simulink model "EDE"  (R2024a)
settings: Solver=VariableStepAuto  StartTime=0.0  StopTime=10  RelTol=1e-3
settings Model: Creator=ansm3  LastModifiedBy=ansm3

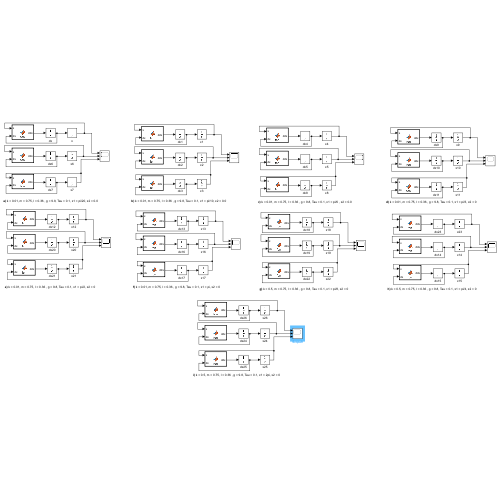
[thumbnail: Simulink's stored preview of the top-level diagram]
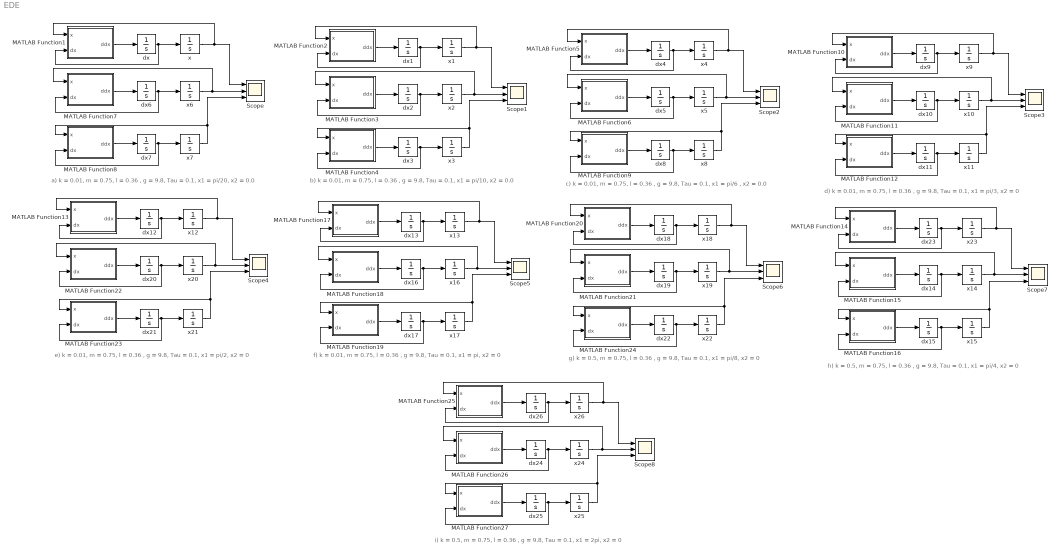
== system EDE ==
  note: a) k = 0.01, m = 0.75, l = 0.36 , g = 9.8, Tau = 0.1, x1 = pi/20, x2 = 0.0
  note: b) k = 0.01, m = 0.75, l = 0.36 , g = 9.8, Tau = 0.1, x1 = pi/10, x2 = 0.0
  note: c) k = 0.01, m = 0.75, l = 0.36 , g = 9.8, Tau = 0.1, x1 = pi/6 , x2 = 0.0
  note: d) k = 0.01, m = 0.75, l = 0.36 , g = 9.8, Tau = 0.1, x1 = pi/3, x2 = 0
  note: e) k = 0.01, m = 0.75, l = 0.36 , g = 9.8, Tau = 0.1, x1 = pi/2, x2 = 0
  note: g) k = 0.5, m = 0.75, l = 0.36 , g = 9.8, Tau = 0.1, x1 = pi/8, x2 = 0
  note: h) k = 0.5, m = 0.75, l = 0.36 , g = 9.8, Tau = 0.1, x1 = pi/4, x2 = 0
  note: f) k = 0.01, m = 0.75, l = 0.36 , g = 9.8, Tau = 0.1, x1 = pi, x2 = 0
  note: i) k = 0.5, m = 0.75, l = 0.36 , g = 9.8, Tau = 0.1, x1 = 2pi, x2 = 0
  MATLAB Function1 : MATLAB Function  TreatAsAtomicUnit=on
  MATLAB Function10 : MATLAB Function  TreatAsAtomicUnit=on
  MATLAB Function11 : MATLAB Function  TreatAsAtomicUnit=on
  MATLAB Function12 : MATLAB Function  TreatAsAtomicUnit=on
  MATLAB Function13 : MATLAB Function  TreatAsAtomicUnit=on
  MATLAB Function14 : MATLAB Function  TreatAsAtomicUnit=on
  MATLAB Function15 : MATLAB Function  TreatAsAtomicUnit=on
  MATLAB Function16 : MATLAB Function  TreatAsAtomicUnit=on
  MATLAB Function17 : MATLAB Function  TreatAsAtomicUnit=on
  MATLAB Function18 : MATLAB Function  TreatAsAtomicUnit=on
  MATLAB Function19 : MATLAB Function  TreatAsAtomicUnit=on
  MATLAB Function2 : MATLAB Function  TreatAsAtomicUnit=on
  MATLAB Function20 : MATLAB Function  TreatAsAtomicUnit=on
  MATLAB Function21 : MATLAB Function  TreatAsAtomicUnit=on
  MATLAB Function22 : MATLAB Function  TreatAsAtomicUnit=on
  MATLAB Function23 : MATLAB Function  TreatAsAtomicUnit=on
  MATLAB Function24 : MATLAB Function  TreatAsAtomicUnit=on
  MATLAB Function25 : MATLAB Function  TreatAsAtomicUnit=on
  MATLAB Function26 : MATLAB Function  TreatAsAtomicUnit=on
  MATLAB Function27 : MATLAB Function  TreatAsAtomicUnit=on
  MATLAB Function3 : MATLAB Function  TreatAsAtomicUnit=on
  MATLAB Function4 : MATLAB Function  TreatAsAtomicUnit=on
  MATLAB Function5 : MATLAB Function  TreatAsAtomicUnit=on
  MATLAB Function6 : MATLAB Function  TreatAsAtomicUnit=on
  MATLAB Function7 : MATLAB Function  TreatAsAtomicUnit=on
  MATLAB Function8 : MATLAB Function  TreatAsAtomicUnit=on
  MATLAB Function9 : MATLAB Function  TreatAsAtomicUnit=on
  Scope{,1..8} (9 alike) : Scope  NumInputPorts=3
  dx{,1..26} (27 alike) : Integrator  ContinuousStateAttributes="\"dx\""
  x : Integrator  InitialCondition=pi/20
  x1 : Integrator  InitialCondition=pi/10
  x10 : Integrator  InitialCondition=pi/3
  x11 : Integrator  InitialCondition=pi/3
  x12 : Integrator  InitialCondition=pi/2
  x13 : Integrator  InitialCondition=pi
  x14 : Integrator  InitialCondition=pi/4
  x15 : Integrator  InitialCondition=pi/4
  x16 : Integrator  InitialCondition=pi
  x17 : Integrator  InitialCondition=pi
  x18 : Integrator  InitialCondition=pi/8
  x19 : Integrator  InitialCondition=pi/8
  x2 : Integrator  InitialCondition=pi/10
  x20 : Integrator  InitialCondition=pi/2
  x21 : Integrator  InitialCondition=pi/2
  x22 : Integrator  InitialCondition=pi/8
  x23 : Integrator  InitialCondition=pi/4
  x24 : Integrator  InitialCondition=2*pi
  x25 : Integrator  InitialCondition=2*pi
  x26 : Integrator  InitialCondition=2*pi
  x3 : Integrator  InitialCondition=pi/10
  x4 : Integrator  InitialCondition=pi/6
  x5 : Integrator  InitialCondition=pi/6
  x6 : Integrator  InitialCondition=pi/20
  x7 : Integrator  InitialCondition=pi/20
  x8 : Integrator  InitialCondition=pi/6
  x9 : Integrator  InitialCondition=pi/3
  wires:
  dx/1 -> x/1, MATLAB Function1/2(dx)
  MATLAB Function1/1(ddx) -> dx/1
  x/1 -> Scope/1, MATLAB Function1/1(x)
  dx6/1 -> x6/1, MATLAB Function7/2(dx)
  MATLAB Function7/1(ddx) -> dx6/1
  x6/1 -> Scope/2, MATLAB Function7/1(x)
  MATLAB Function8/1(ddx) -> dx7/1
  dx7/1 -> x7/1, MATLAB Function8/2(dx)
  x7/1 -> Scope/3, MATLAB Function8/1(x)
  x2/1 -> Scope1/2, MATLAB Function3/1(x)
  MATLAB Function3/1(ddx) -> dx2/1
  dx2/1 -> x2/1, MATLAB Function3/2(dx)
  MATLAB Function4/1(ddx) -> dx3/1
  dx3/1 -> x3/1, MATLAB Function4/2(dx)
  dx1/1 -> x1/1, MATLAB Function2/2(dx)
  x3/1 -> Scope1/3, MATLAB Function4/1(x)
  x1/1 -> Scope1/1, MATLAB Function2/1(x)
  MATLAB Function2/1(ddx) -> dx1/1
  dx8/1 -> x8/1, MATLAB Function9/2(dx)
  dx5/1 -> x5/1, MATLAB Function6/2(dx)
  MATLAB Function9/1(ddx) -> dx8/1
  MATLAB Function6/1(ddx) -> dx5/1
  dx4/1 -> x4/1, MATLAB Function5/2(dx)
  x8/1 -> Scope2/3, MATLAB Function9/1(x)
  MATLAB Function5/1(ddx) -> dx4/1
  x4/1 -> Scope2/1, MATLAB Function5/1(x)
  x5/1 -> Scope2/2, MATLAB Function6/1(x)
  x11/1 -> Scope3/3, MATLAB Function12/1(x)
  x9/1 -> Scope3/1, MATLAB Function10/1(x)
  MATLAB Function10/1(ddx) -> dx9/1
  x10/1 -> Scope3/2, MATLAB Function11/1(x)
  dx9/1 -> x9/1, MATLAB Function10/2(dx)
  dx11/1 -> x11/1, MATLAB Function12/2(dx)
  MATLAB Function11/1(ddx) -> dx10/1
  MATLAB Function12/1(ddx) -> dx11/1
  dx10/1 -> x10/1, MATLAB Function11/2(dx)
  x20/1 -> Scope4/2, MATLAB Function22/1(x)
  dx14/1 -> x14/1, MATLAB Function15/2(dx)
  MATLAB Function15/1(ddx) -> dx14/1
  dx15/1 -> x15/1, MATLAB Function16/2(dx)
  MATLAB Function16/1(ddx) -> dx15/1
  x15/1 -> Scope7/3, MATLAB Function16/1(x)
  x14/1 -> Scope7/2, MATLAB Function15/1(x)
  MATLAB Function14/1(ddx) -> dx23/1
  MATLAB Function20/1(ddx) -> dx18/1
  dx16/1 -> x16/1, MATLAB Function18/2(dx)
  MATLAB Function19/1(ddx) -> dx17/1
  x23/1 -> Scope7/1, MATLAB Function14/1(x)
  dx23/1 -> x23/1, MATLAB Function14/2(dx)
  MATLAB Function18/1(ddx) -> dx16/1
  dx13/1 -> x13/1, MATLAB Function17/2(dx)
  x17/1 -> Scope5/3, MATLAB Function19/1(x)
  x19/1 -> Scope6/2, MATLAB Function21/1(x)
  MATLAB Function17/1(ddx) -> dx13/1
  x13/1 -> Scope5/1, MATLAB Function17/1(x)
  x22/1 -> Scope6/3, MATLAB Function24/1(x)
  MATLAB Function21/1(ddx) -> dx19/1
  MATLAB Function24/1(ddx) -> dx22/1
  MATLAB Function22/1(ddx) -> dx20/1
  dx20/1 -> x20/1, MATLAB Function22/2(dx)
  dx17/1 -> x17/1, MATLAB Function19/2(dx)
  dx21/1 -> x21/1, MATLAB Function23/2(dx)
  MATLAB Function23/1(ddx) -> dx21/1
  x16/1 -> Scope5/2, MATLAB Function18/1(x)
  dx12/1 -> x12/1, MATLAB Function13/2(dx)
  dx22/1 -> x22/1, MATLAB Function24/2(dx)
  x21/1 -> Scope4/3, MATLAB Function23/1(x)
  x18/1 -> Scope6/1, MATLAB Function20/1(x)
  MATLAB Function13/1(ddx) -> dx12/1
  dx19/1 -> x19/1, MATLAB Function21/2(dx)
  x12/1 -> Scope4/1, MATLAB Function13/1(x)
  dx18/1 -> x18/1, MATLAB Function20/2(dx)
  MATLAB Function27/1(ddx) -> dx25/1
  MATLAB Function26/1(ddx) -> dx24/1
  dx24/1 -> x24/1, MATLAB Function26/2(dx)
  dx25/1 -> x25/1, MATLAB Function27/2(dx)
  x25/1 -> Scope8/3, MATLAB Function27/1(x)
  dx26/1 -> x26/1, MATLAB Function25/2(dx)
  x26/1 -> Scope8/1, MATLAB Function25/1(x)
  x24/1 -> Scope8/2, MATLAB Function26/1(x)
  MATLAB Function25/1(ddx) -> dx26/1

== matlab function EDE/MATLAB Function13 ==
  data: x input; ddx output; dx input
function ddx = fcn(x, dx)

k=0.01;
l=0.36;
g=9.8;
a=l/2;

m=0.75;
J=(4/3)*(m*a^2);
tao=0.1;

ddx=(tao/J) - ((k*dx)/J) - ((m*g*a*x)/J);

== matlab function EDE/MATLAB Function14 ==
  data: x input; ddx output; dx input
function ddx = fcn(x, dx)

k=0.5;
l=0.36;
g=9.8;
a=l/2;

m=0.75;
J=(4/3)*(m*a^2);
tao=0.1;

ddx=(tao/J) - ((k*dx)/J) - ((m*g*a*x)/J);

== matlab function EDE/MATLAB Function15 ==
  data: x input; ddx output; dx input
function ddx = fcn(x, dx)

k=0.5;
l=0.36;
g=9.8;
a=l/2;

m=0.75;
J=(4/3)*(m*a^2);
tao=0.1;

ddx=(tao/J) - ((k*dx)/J) - ((m*g*a*sin(x))/J);

== matlab function EDE/MATLAB Function16 ==
  data: x input; ddx output; dx input
function ddx = fcn(x, dx)

k=0.5;
l=0.36;
g=9.8;
a=l/2;

m=0.75;
J=(4/3)*(m*a^2);
tao=0.1;

ddx=(tao/J) - ((k*dx)/J) - ((m*g*a*cos(x))/J);

== matlab function EDE/MATLAB Function17 ==
  data: x input; ddx output; dx input
function ddx = fcn(x, dx)

k=0.01;
l=0.36;
g=9.8;
a=l/2;

m=0.75;
J=(4/3)*(m*a^2);
tao=0.1;

ddx=(tao/J) - ((k*dx)/J) - ((m*g*a*x)/J);

== matlab function EDE/MATLAB Function18 ==
  data: x input; ddx output; dx input
function ddx = fcn(x, dx)

k=0.01;
l=0.36;
g=9.8;
a=l/2;

m=0.75;
J=(4/3)*(m*a^2);
tao=0.1;

ddx=(tao/J) - ((k*dx)/J) - ((m*g*a*sin(x))/J);

== matlab function EDE/MATLAB Function19 ==
  data: x input; ddx output; dx input
function ddx = fcn(x, dx)

k=0.01;
l=0.36;
g=9.8;
a=l/2;

m=0.75;
J=(4/3)*(m*a^2);
tao=0.1;

ddx=(tao/J) - ((k*dx)/J) - ((m*g*a*cos(x))/J);

== matlab function EDE/MATLAB Function2 ==
  data: x input; ddx output; dx input
function ddx = fcn(x, dx)

k=0.01;
l=0.36;
g=9.8;
a=l/2;

m=0.75;
J=(4/3)*(m*a^2);
tao=0.1;

ddx=(tao/J) - ((k*dx)/J) - ((m*g*a*x)/J);

== matlab function EDE/MATLAB Function20 ==
  data: x input; ddx output; dx input
function ddx = fcn(x, dx)

k=0.5;
l=0.36;
g=9.8;
a=l/2;

m=0.75;
J=(4/3)*(m*a^2);
tao=0.1;

ddx=(tao/J) - ((k*dx)/J) - ((m*g*a*x)/J);

== matlab function EDE/MATLAB Function21 ==
  data: x input; ddx output; dx input
function ddx = fcn(x, dx)

k=0.5;
l=0.36;
g=9.8;
a=l/2;

m=0.75;
J=(4/3)*(m*a^2);
tao=0.1;

ddx=(tao/J) - ((k*dx)/J) - ((m*g*a*sin(x))/J);

== matlab function EDE/MATLAB Function22 ==
  data: x input; ddx output; dx input
function ddx = fcn(x, dx)

k=0.01;
l=0.36;
g=9.8;
a=l/2;

m=0.75;
J=(4/3)*(m*a^2);
tao=0.1;

ddx=(tao/J) - ((k*dx)/J) - ((m*g*a*sin(x))/J);

== matlab function EDE/MATLAB Function23 ==
  data: x input; ddx output; dx input
function ddx = fcn(x, dx)

k=0.01;
l=0.36;
g=9.8;
a=l/2;

m=0.75;
J=(4/3)*(m*a^2);
tao=0.1;

ddx=(tao/J) - ((k*dx)/J) - ((m*g*a*cos(x))/J);

== matlab function EDE/MATLAB Function24 ==
  data: x input; ddx output; dx input
function ddx = fcn(x, dx)

k=0.5;
l=0.36;
g=9.8;
a=l/2;

m=0.75;
J=(4/3)*(m*a^2);
tao=0.1;

ddx=(tao/J) - ((k*dx)/J) - ((m*g*a*cos(x))/J);

== matlab function EDE/MATLAB Function25 ==
  data: x input; ddx output; dx input
function ddx = fcn(x, dx)

k=0.5;
l=0.36;
g=9.8;
a=l/2;

m=0.75;
J=(4/3)*(m*a^2);
tao=0.1;

ddx=(tao/J) - ((k*dx)/J) - ((m*g*a*x)/J);

== matlab function EDE/MATLAB Function26 ==
  data: x input; ddx output; dx input
function ddx = fcn(x, dx)

k=0.5;
l=0.36;
g=9.8;
a=l/2;

m=0.75;
J=(4/3)*(m*a^2);
tao=0.1;

ddx=(tao/J) - ((k*dx)/J) - ((m*g*a*sin(x))/J);

== matlab function EDE/MATLAB Function27 ==
  data: x input; ddx output; dx input
function ddx = fcn(x, dx)

k=0.5;
l=0.36;
g=9.8;
a=l/2;

m=0.75;
J=(4/3)*(m*a^2);
tao=0.1;

ddx=(tao/J) - ((k*dx)/J) - ((m*g*a*cos(x))/J);

== matlab function EDE/MATLAB Function3 ==
  data: x input; ddx output; dx input
function ddx = fcn(x, dx)

k=0.01;
l=0.36;
g=9.8;
a=l/2;

m=0.75;
J=(4/3)*(m*a^2);
tao=0.1;

ddx=(tao/J) - ((k*dx)/J) - ((m*g*a*sin(x))/J);

== matlab function EDE/MATLAB Function4 ==
  data: x input; ddx output; dx input
function ddx = fcn(x, dx)

k=0.01;
l=0.36;
g=9.8;
a=l/2;

m=0.75;
J=(4/3)*(m*a^2);
tao=0.1;

ddx=(tao/J) - ((k*dx)/J) - ((m*g*a*cos(x))/J);

== matlab function EDE/MATLAB Function5 ==
  data: x input; ddx output; dx input
function ddx = fcn(x, dx)

k=0.01;
l=0.36;
g=9.8;
a=l/2;

m=0.75;
J=(4/3)*(m*a^2);
tao=0.1;

ddx=(tao/J) - ((k*dx)/J) - ((m*g*a*x)/J);

== matlab function EDE/MATLAB Function6 ==
  data: x input; ddx output; dx input
function ddx = fcn(x, dx)

k=0.01;
l=0.36;
g=9.8;
a=l/2;

m=0.75;
J=(4/3)*(m*a^2);
tao=0.1;

ddx=(tao/J) - ((k*dx)/J) - ((m*g*a*sin(x))/J);

== matlab function EDE/MATLAB Function7 ==
  data: x input; ddx output; dx input
function ddx = fcn(x, dx)

k=0.01;
l=0.36;
g=9.8;
a=l/2;

m=0.75;
J=(4/3)*(m*a^2);
tao=0.1;

ddx=(tao/J) - ((k*dx)/J) - ((m*g*a*sin(x))/J);

== matlab function EDE/MATLAB Function8 ==
  data: x input; ddx output; dx input
function ddx = fcn(x, dx)

k=0.01;
l=0.36;
g=9.8;
a=l/2;

m=0.75;
J=(4/3)*(m*a^2);
tao=0.1;

ddx=(tao/J) - ((k*dx)/J) - ((m*g*a*cos(x))/J);

== matlab function EDE/MATLAB Function9 ==
  data: x input; ddx output; dx input
function ddx = fcn(x, dx)

k=0.01;
l=0.36;
g=9.8;
a=l/2;

m=0.75;
J=(4/3)*(m*a^2);
tao=0.1;

ddx=(tao/J) - ((k*dx)/J) - ((m*g*a*cos(x))/J);

== matlab function EDE/MATLAB Function1 ==
  data: x input; ddx output; dx input
function ddx = fcn(x, dx)

k=0.01;
l=0.36;
g=9.8;
a=l/2;

m=0.75;
J=(4/3)*(m*a^2);
tao=0.1;

ddx=(tao/J) - ((k*dx)/J) - ((m*g*a*x)/J);

== matlab function EDE/MATLAB Function10 ==
  data: x input; ddx output; dx input
function ddx = fcn(x, dx)

k=0.01;
l=0.36;
g=9.8;
a=l/2;

m=0.75;
J=(4/3)*(m*a^2);
tao=0.1;

ddx=(tao/J) - ((k*dx)/J) - ((m*g*a*x)/J);

== matlab function EDE/MATLAB Function11 ==
  data: x input; ddx output; dx input
function ddx = fcn(x, dx)

k=0.01;
l=0.36;
g=9.8;
a=l/2;

m=0.75;
J=(4/3)*(m*a^2);
tao=0.1;

ddx=(tao/J) - ((k*dx)/J) - ((m*g*a*sin(x))/J);

== matlab function EDE/MATLAB Function12 ==
  data: x input; ddx output; dx input
function ddx = fcn(x, dx)

k=0.01;
l=0.36;
g=9.8;
a=l/2;

m=0.75;
J=(4/3)*(m*a^2);
tao=0.1;

ddx=(tao/J) - ((k*dx)/J) - ((m*g*a*cos(x))/J);
